simulink model "bla"  (R2023b)
settings: Solver=VariableStepAuto  StartTime=0.0  StopTime=10.0  RelTol=1e-3
undefined symbols (not defined in the file or in its folder): Bat, boost, ccm_mpp_reg_param, ccm_reg_param, Ci, dcm_mpp_reg_param, dcm_reg_param, m0_ccm, mppt_my3, pv_data, pv_eq, Ramp, sim_op, Tmfc, Ubat_CV_limit, Upv_ref
libraries: spsSeriesRLCBranchLib x5, spsCurrentMeasurementLib x2, spsVoltageMeasurementLib x2, spsControlledVoltageSourceLib x1, spsDiodeLib x1, spsControlledCurrentSourceLib x1, spsBistableLib x1, slpidlib x1, spsIdealSwitchLib x1
settings Model: Creator=teo  LastModifiedBy=teo

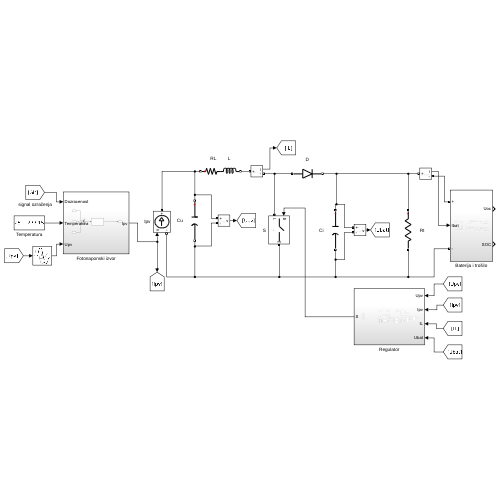
[thumbnail: Simulink's stored preview of the top-level diagram]
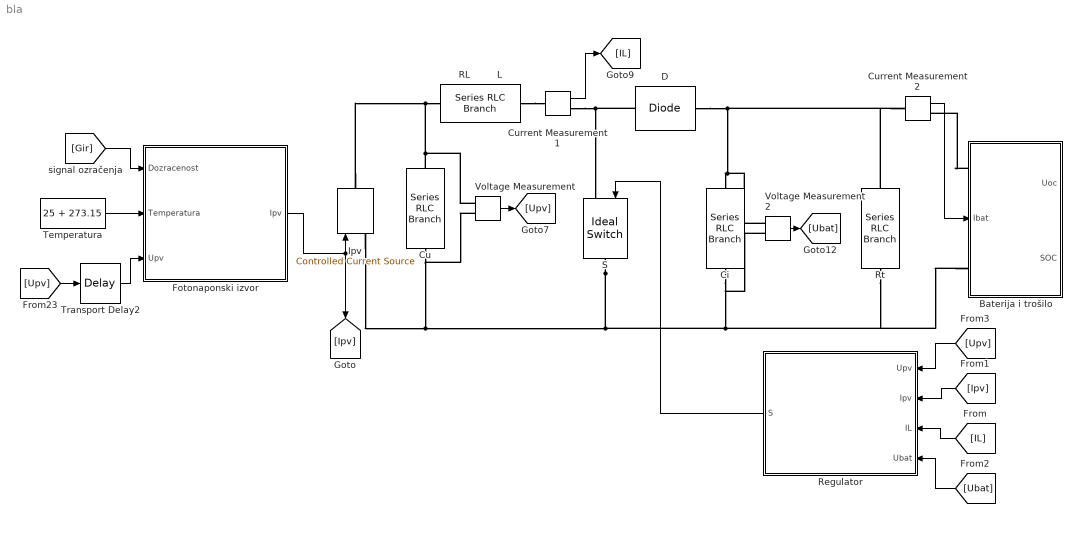
== system bla ==
  Baterija i trošilo : Subsystem
      settings: PortSchema="{\"entries\":[{\"content\":{\"sides\":[{\"content\":{\"connectorIds\":[\"LConn1\",\"In1\",\"LConn2\"]},\"type\":\"ConnectorPlacement.EquallySpacedRectSide\",\"uuid\":\"36a151cb-ade8-4d77-9227-5d94720a867f\"},{\"content\":{\"connectorIds\":[\"Out1\",\"Out2\"],\"side\":\"RIGHT\"},\"type\":\"ConnectorPlacement.EquallySpacedRectSide\",\"uuid\":\"e273b59b-5ac5-431a-9422-aa1eb85d6b42\"},{\"content\":{\"side\":\"TOP\"},\"type\":\"ConnectorPlacement.EquallySpacedRectSide\",\"uuid\":\"963da400-5a20-4c48-ad4c-e087b1b0be12\"}]},\"type\":\"ConnectorPlacement.EquallySpacedConnector\",\"uuid\":\"3f6c7281-abab-4595-a869-b172f12b4791\"}],\"packageUris\":[\"http://schema.mathworks.com/mf0/Connector/R2020b\"],\"version\":\"1.0\"}"
  Ci : spsSeriesRLCBranchLib/Series RLC Branch  LConnTagsString=__new0  RConnTagsString=__new0  BranchType=C  Resistance=0.001  Inductance=1e-3  SetiL0=off  InitialCurrent=0  Capacitance=boost.Ci  Setx0=on  InitialVoltage=sim_op.Ubat0  Measurements=None
  Cu : spsSeriesRLCBranchLib/Series RLC Branch  LConnTagsString=__new0  RConnTagsString=__new0  BranchType=C  Resistance=0.001  Inductance=1e-3  SetiL0=off  InitialCurrent=0  Capacitance=boost.Cu  Setx0=on  InitialVoltage=sim_op.Upv0  Measurements=None
  Current Measurement1 : spsCurrentMeasurementLib/Current Measurement  PhasorSimulation=off  OutputType=Complex  PSBequivalent=0
  Current Measurement2 : spsCurrentMeasurementLib/Current Measurement  PhasorSimulation=off  OutputType=Complex  PSBequivalent=0
  D : spsDiodeLib/Diode  Ron=0  Lon=0  Vf=0  IC=0  UseSnubber=0  Rs=0  Cs=0  Measurements=off
  Fotonaponski izvor : Subsystem
  Ipv : spsControlledCurrentSourceLib/Controlled Current Source  Initialize=on  Source_Type=DC  Amplitude=0  Phase=0  Frequency=0  Measurements=None
  RL         L : spsSeriesRLCBranchLib/Series RLC Branch  LConnTagsString=__new0  RConnTagsString=__new0  BranchType=RL  Resistance=boost.RL  Inductance=boost.L  SetiL0=off  InitialCurrent=stepp.ir01  Capacitance=1e-6  Setx0=off  InitialVoltage=0  Measurements=None
  Regulator : Subsystem
  Rt : spsSeriesRLCBranchLib/Series RLC Branch  LConnTagsString=__new0  RConnTagsString=__new0  BranchType=R  Resistance=boost.Rt  Inductance=1e-3  SetiL0=off  InitialCurrent=0  Capacitance=Ci  Setx0=off  InitialVoltage=0  Measurements=None
  S : spsIdealSwitchLib/Ideal Switch  Ron=0  Lon=0  IC=0  Rs=0  Cs=0  Measurements=off
  Temperatura : Constant  Value=25 + 273.15
  Transport Delay2 : TransportDelay  DelayTime=0.0001  BufferSize=4024
  Voltage Measurement : spsVoltageMeasurementLib/Voltage Measurement  PhasorSimulation=off  OutputType=Complex  PSBequivalent=0
  Voltage Measurement2 : spsVoltageMeasurementLib/Voltage Measurement  PhasorSimulation=off  OutputType=Complex  PSBequivalent=0
  wires:
  Voltage Measurement2/1 -> [Ubat]
  Current Measurement1/1 -> [IL]
  [Gir] -> Fotonaponski izvor/1(Dozracenost)
  Temperatura/1 -> Fotonaponski izvor/2(Temperatura)
  Regulator/1(S) -> S/1
  Fotonaponski izvor/1(Ipv) -> Ipv/1, [Ipv]
  [Upv] -> Transport Delay2/1
  Transport Delay2/1 -> Fotonaponski izvor/3(Upv)
  Voltage Measurement/1 -> [Upv]
  Current Measurement2/1 -> Baterija i trošilo/1(Ibat)
  [IL] -> Regulator/3(IL)
  [Ipv] -> Regulator/2(Ipv)
  [Ubat] -> Regulator/4(Ubat)
  [Upv] -> Regulator/1(Upv)
  connections:
  S/RConn1 -- Baterija i trošilo/LConn2 -- Rt/RConn1 -- Ci/RConn1 -- Voltage Measurement2/LConn2 -- Ipv/LConn1 -- Voltage Measurement/LConn2 -- Cu/RConn1
  D/RConn1 -- Current Measurement2/LConn1 -- Rt/LConn1 -- Voltage Measurement2/LConn1 -- Ci/LConn1
  Cu/LConn1 -- Voltage Measurement/LConn1 -- Ipv/RConn1 -- RL         L/LConn1
  Current Measurement1/RConn1 -- D/LConn1 -- S/LConn1
  Baterija i trošilo/LConn1 -- Current Measurement2/RConn1
  RL         L/RConn1 -- Current Measurement1/LConn1

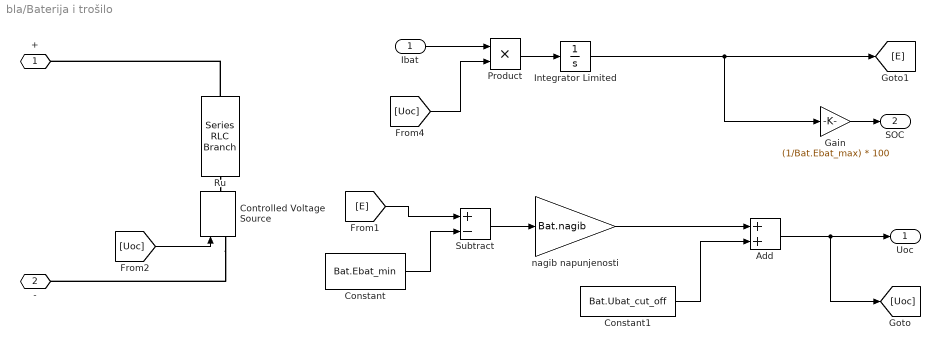
== system bla/Baterija i trošilo ==
  Ibat : Inport
  Add : Sum
  Constant : Constant  Value=Bat.Ebat_min
  Constant1 : Constant  Value=Bat.Ubat_cut_off
  Controlled Voltage Source : spsControlledVoltageSourceLib/Controlled Voltage Source  Initialize=on  Source_Type=DC  Amplitude=sim_op.Ubat0  Phase=0  Frequency=0  Measurements=None
  Gain : Gain  Gain=(1/Bat.Ebat_max) * 100
  Integrator Limited : Integrator  InitialCondition=sim_op.E0  LimitOutput=on  UpperSaturationLimit=Bat.Ebat_max  LowerSaturationLimit=Bat.Ebat_min
  Product : Product
  Ru : spsSeriesRLCBranchLib/Series RLC Branch  LConnTagsString=__new0  RConnTagsString=__new0  BranchType=R  Resistance=boost.Ru  Inductance=1e-3  SetiL0=off  InitialCurrent=0  Capacitance=Ci  Setx0=off  InitialVoltage=0  Measurements=None
  Subtract : Sum  Inputs=+-
  nagib napunjenosti : Gain  Gain=Bat.nagib
  + : PMIOPort  Side=Left
  - : PMIOPort  Port=2  Side=Left
  Uoc : Outport
  SOC : Outport  Port=2
  wires:
  Subtract/1 -> nagib napunjenosti/1
  Constant/1 -> Subtract/2
  nagib napunjenosti/1 -> Add/1
  Constant1/1 -> Add/2
  Integrator Limited/1 -> Gain/1, [E]
  [Uoc] -> Product/2
  Product/1 -> Integrator Limited/1
  Ibat/1 -> Product/1
  [E] -> Subtract/1
  [Uoc] -> Controlled Voltage Source/1
  Gain/1 -> SOC/1
  Add/1 -> Uoc/1, [Uoc]
  connections:
  Controlled Voltage Source/LConn1 -- -/RConn1
  Ru/RConn1 -- Controlled Voltage Source/RConn1
  Ru/LConn1 -- +/RConn1

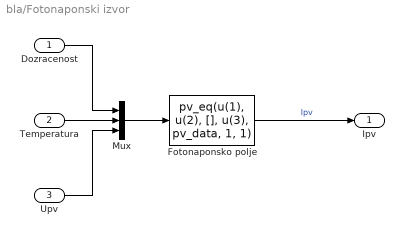
== system bla/Fotonaponski izvor ==
  Dozracenost : Inport
  Temperatura : Inport  Port=2
  Upv : Inport  Port=3
  Fotonaponsko polje : MATLABFcn  MATLABFcn=pv_eq(u(1), u(2), [], u(3), pv_data, 1, 1)  OutputDimensions=1
  Mux : Mux  Inputs=3
  Ipv : Outport
  wires:
  Fotonaponsko polje/1 -> Ipv/1  "Ipv"
  Mux/1 -> Fotonaponsko polje/1
  Dozracenost/1 -> Mux/1
  Temperatura/1 -> Mux/2
  Upv/1 -> Mux/3

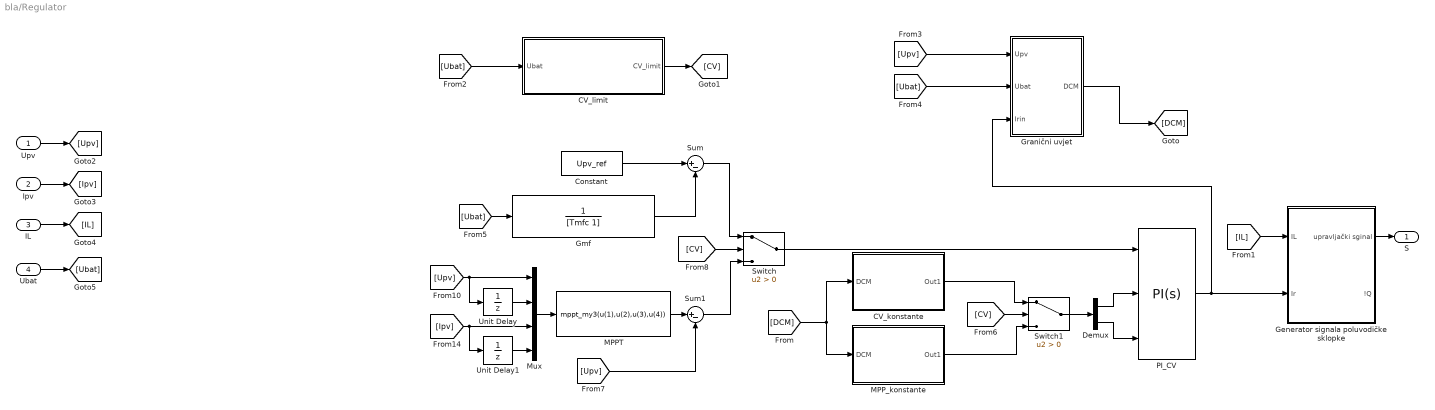
== system bla/Regulator ==
  Upv : Inport
  Ipv : Inport  Port=2
  IL : Inport  Port=3
  Ubat : Inport  Port=4
  CV_konstante : Subsystem
  CV_limit : Subsystem
  Constant : Constant  Value=Upv_ref
  Demux : Demux  Outputs=2
  Generator signala poluvodičke sklopke : Subsystem
  Gmf : TransferFcn  Numerator=1  Denominator=[Tmfc 1]
  Granični uvjet : Subsystem
  MPPT : MATLABFcn  MATLABFcn=mppt_my3(u(1),u(2),u(3),u(4))
  MPP_konstante : Subsystem
  Mux : Mux
  PI_CV : slpidlib/PID Controller  Controller=PI  Form=Parallel  TimeDomain=Continuous-time  UseExternalTs=off  SampleTime=-1  IntegratorMethod=Forward Euler  FilterMethod=Forward Euler  ControllerParametersSource=external  P=ccm_mpp_reg_param.KR  I=ccm_mpp_reg_param.KR/ccm_mpp_reg_param.Ti  UseKiTs=off  D=0  N=100  UseFilter=on  TunerSelectOption=Transfer Function Based (PID Tuner App)  InitialConditionSource=internal  InitialConditionForIntegrator=0  InitialConditionForFilter=0  DifferentiatorICPrevScaledInput=0  ExternalReset=none  TrackingMode=off  Kt=1  LimitOutput=on  SatLimitsSource=internal  UpperSaturationLimit=2  LowerSaturationLimit=-2  LinearizeAsGain=off  AntiWindupMode=clamping  Kb=1  LimitIntegrator=off  UpperIntegratorSaturationLimit=inf  LowerIntegratorSaturationLimit=-inf  POutMin=[]  POutMax=[]  IOutMin=[]  IOutMax=[]  DOutMin=[]  DOutMax=[]  NOutMin=[]  NOutMax=[]  SumOutMin=[]  SumOutMax=[]  SaturationOutMin=[]  SaturationOutMax=[]  PParamMin=[]  PParamMax=[]  IParamMin=[]  IParamMax=[]  DParamMin=[]  DParamMax=[]  NParamMin=[]  NParamMax=[]  KbParamMin=[]  KbParamMax=[]  KtParamMin=[]  KtParamMax=[]  KbOutMin=[]  KbOutMax=[]  KtOutMin=[]  KtOutMax=[]  IntegratorOutMin=[]  IntegratorOutMax=[]  FilterOutMin=[]  FilterOutMax=[]  SumI1OutMin=[]  SumI1OutMax=[]  SumI2OutMin=[]  SumI2OutMax=[]  SumI3OutMin=[]  SumI3OutMax=[]  SumI4OutMin=[]  SumI4OutMax=[]  SumDOutMin=[]  SumDOutMax=[]  DifferentiatorOutMin=[]  DifferentiatorOutMax=[]  FilterDiffOutCoefMin=[]  FilterDiffOutCoefMax=[]  ReciprocalOutMin=[]  ReciprocalOutMax=[]  SumDenOutMin=[]  SumDenOutMax=[]  SumNumOutMin=[]  SumNumOutMax=[]  DivideOutMin=[]  DivideOutMax=[]  UdiffTsProdOutMin=[]  UdiffTsProdOutMax=[]  NTsProdOutMin=[]  NTsProdOutMax=[]  UintegralTsProdOutMin=[]  UintegralTsProdOutMax=[]  UngainTsProdOutMin=[]  UngainTsProdOutMax=[]  ClampingZeroOutDataTypeStr=Inherit: Inherit via back propagation  ClampingZeroOutMin=[]  ClampingZeroOutMax=[]  FilterDenConstantOutDataTypeStr=Inherit: Inherit via back propagation  FilterDenConstantOutMin=[]  FilterDenConstantOutMax=[]  PCopyOutDataTypeStr=Inherit: Inherit via back propagation  PCopyOutMin=[]  PCopyOutMax=[]  NCopyOutDataTypeStr=Inherit: Inherit via back propagation  NCopyOutMin=[]  NCopyOutMax=[]  IntegratorContinuousStateAttributes=''  IntegratorStateMustResolveToSignalObject=off  IntegratorRTWStateStorageClass=Auto  FilterContinuousStateAttributes=''  FilterStateMustResolveToSignalObject=off  FilterRTWStateStorageClass=Auto  ParallelPVariant=ExternalParameters  IdealPVariant=Disabled  IVariant=ExternalParameters  DVariant=Disabled  IntegratorVariant=Continuous  SatVariant=Enabled  AWVariant=ContClampingParallel  PCopyVariant=Disabled  TRVariant=Disabled  FdbkBlocksVariant=Forward  IdealPFdbkVariant=Disabled  SatFdbkVariant=Disabled  DerivativeFilterVariant=Disabled  NVariant=Disabled  NCopyVariant=Disabled_SignalSpec  FilterICVariant=Disabled  IntegratorICVariant=InternalICs  ExternalResetVariant=Disabled  TRSumVariant=Passthrough  SumFdbkVariant=Disabled  SumVariant=Sum_PI  TsampFilterVariant=InternalTs  TsampNgainVariant=Passthrough  TsampIntegralVariant=Disabled_SignalSpec  ExternalSaturationOutDataTypeStr=Inherit: Same as second input
  Sum : Sum  Inputs=|+-
  Sum1 : Sum  Inputs=|+-
  Switch : Switch  Criteria=u2 > Threshold  SaturateOnIntegerOverflow=off  InputSameDT=off
  Switch1 : Switch  Criteria=u2 > Threshold  SaturateOnIntegerOverflow=off  InputSameDT=off
  Unit Delay : UnitDelay  SampleTime=-1  HasFrameUpgradeWarning=on
  Unit Delay1 : UnitDelay  SampleTime=-1  HasFrameUpgradeWarning=on
  S : Outport
  wires:
  Switch1/1 -> Demux/1
  Demux/1 -> PI_CV/2
  Demux/2 -> PI_CV/3
  Generator signala poluvodičke sklopke/1(upravljački sginal) -> S/1
  Upv/1 -> [Upv]
  Ipv/1 -> [Ipv]
  Ubat/1 -> [Ubat]
  IL/1 -> [IL]
  Granični uvjet/1(DCM) -> [DCM]
  [Ubat] -> Granični uvjet/2(Ubat)
  PI_CV/1 -> Generator signala poluvodičke sklopke/2(Ir), Granični uvjet/3(Irin)
  [IL] -> Generator signala poluvodičke sklopke/1(IL)
  [Ubat] -> Gmf/1
  Constant/1 -> Sum/1
  Gmf/1 -> Sum/2
  Unit Delay1/1 -> Mux/4
  Unit Delay/1 -> Mux/2
  MPPT/1 -> Sum1/1
  [Upv] -> Sum1/2
  Mux/1 -> MPPT/1
  [Upv] -> Unit Delay/1, Mux/1
  [Ipv] -> Unit Delay1/1, Mux/3
  CV_konstante/1(Out1) -> Switch1/1
  MPP_konstante/1(Out1) -> Switch1/3
  [DCM] -> MPP_konstante/1(DCM), CV_konstante/1(DCM)
  [Ubat] -> CV_limit/1(Ubat)
  [Upv] -> Granični uvjet/1(Upv)
  CV_limit/1(CV_limit) -> [CV]
  [CV] -> Switch1/2
  [CV] -> Switch/2
  Switch/1 -> PI_CV/1
  Sum/1 -> Switch/1
  Sum1/1 -> Switch/3

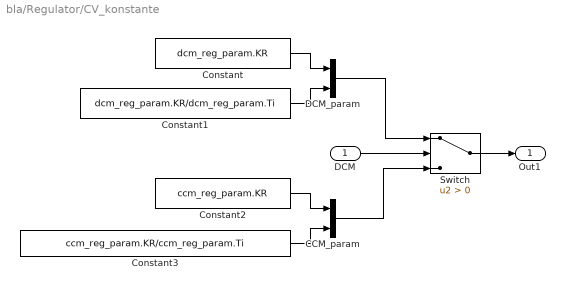
== system bla/Regulator/CV_konstante ==
  DCM : Inport
  CCM_param : Mux  Inputs=2
  Constant : Constant  Value=dcm_reg_param.KR
  Constant1 : Constant  Value=dcm_reg_param.KR/dcm_reg_param.Ti
  Constant2 : Constant  Value=ccm_reg_param.KR
  Constant3 : Constant  Value=ccm_reg_param.KR/ccm_reg_param.Ti
  DCM_param : Mux  Inputs=2
  Switch : Switch  Criteria=u2 > Threshold  SaturateOnIntegerOverflow=off  InputSameDT=off
  Out1 : Outport
  wires:
  Constant/1 -> DCM_param/1
  Constant1/1 -> DCM_param/2
  DCM_param/1 -> Switch/1
  Constant2/1 -> CCM_param/1
  Constant3/1 -> CCM_param/2
  CCM_param/1 -> Switch/3
  Switch/1 -> Out1/1
  DCM/1 -> Switch/2

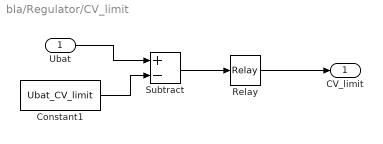
== system bla/Regulator/CV_limit ==
  Ubat : Inport
  Constant1 : Constant  Value=Ubat_CV_limit
  Relay : Relay  OnSwitchValue=0  OffSwitchValue=-0.5
  Subtract : Sum  Inputs=+-
  CV_limit : Outport
  wires:
  Constant1/1 -> Subtract/2
  Subtract/1 -> Relay/1
  Relay/1 -> CV_limit/1
  Ubat/1 -> Subtract/1

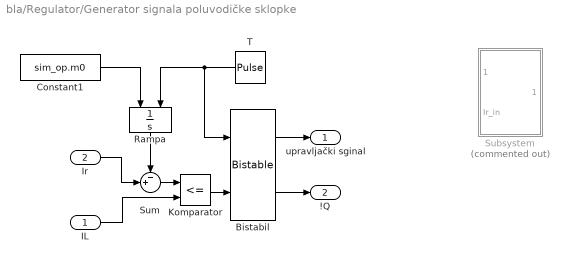
== system bla/Regulator/Generator signala poluvodičke sklopke ==
  IL : Inport
  Ir : Inport  Port=2
  Bistabil : spsBistableLib/Bistable  Qpriority=Set  ic=0  Ts=0
      settings: LibrarySourceBlock=sps_lib/Control/Bistable
  Constant1 : Constant  Value=sim_op.m0
  Komparator : RelationalOperator  Operator=<=  OutDataTypeStr=boolean  RndMeth=Simplest  InputSameDT=off
  Rampa : Integrator  ExternalReset=rising
  Subsystem : Subsystem  Commented=on
  Sum : Sum  Inputs=-+|
  T : DiscretePulseGenerator  PulseType=Time based  Period=boost.T
  upravljački sginal : Outport
  !Q : Outport  Port=2
  wires:
  Komparator/1 -> Bistabil/2
  Bistabil/2 -> !Q/1
  Bistabil/1 -> upravljački sginal/1
  IL/1 -> Komparator/2
  Sum/1 -> Komparator/1
  Ir/1 -> Sum/2
  Rampa/1 -> Sum/1
  T/1 -> Bistabil/1, Rampa/2
  Constant1/1 -> Rampa/1

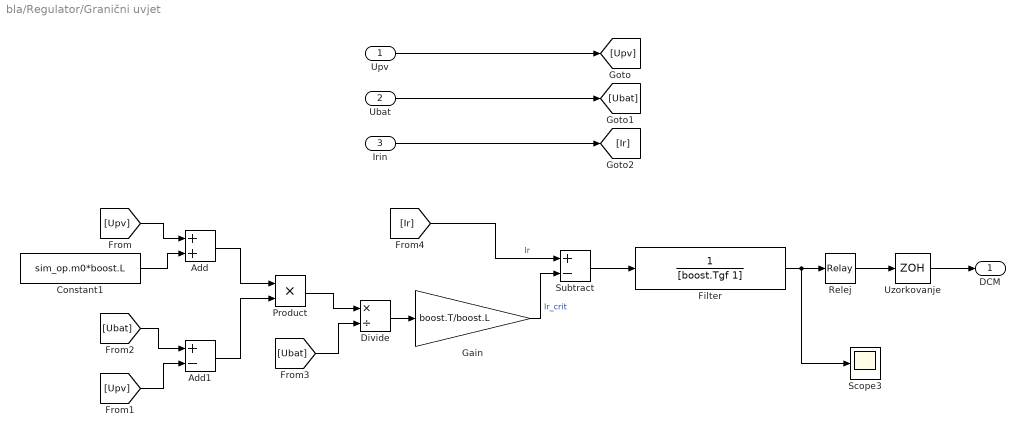
== system bla/Regulator/Granični uvjet ==
  Upv : Inport
  Ubat : Inport  Port=2
  Irin : Inport  Port=3
  Add : Sum
  Add1 : Sum  Inputs=+-
  Constant1 : Constant  Value=sim_op.m0*boost.L
  Divide : Product  Inputs=*/
  Filter : TransferFcn  Numerator=1  Denominator=[boost.Tgf 1]
  Gain : Gain  Gain=boost.T/boost.L
  Product : Product
  Relej : Relay  OnSwitchValue=0.01  OffSwitchValue=-0.01  OnOutputValue=0  OffOutputValue=1
  Scope3 : Scope
  Subtract : Sum  Inputs=+-
  Uzorkovanje : ZeroOrderHold  SampleTime=0.001
  DCM : Outport
  wires:
  Product/1 -> Divide/1
  Constant1/1 -> Add/2
  Add/1 -> Product/1
  Add1/1 -> Product/2
  Divide/1 -> Gain/1
  [Upv] -> Add/1
  [Upv] -> Add1/2
  [Ubat] -> Add1/1
  [Ubat] -> Divide/2
  Gain/1 -> Subtract/2  "Ir_crit"
  [Ir] -> Subtract/1  "Ir"
  Relej/1 -> Uzorkovanje/1
  Upv/1 -> [Upv]
  Ubat/1 -> [Ubat]
  Irin/1 -> [Ir]
  Subtract/1 -> Filter/1
  Filter/1 -> Scope3/1, Relej/1
  Uzorkovanje/1 -> DCM/1

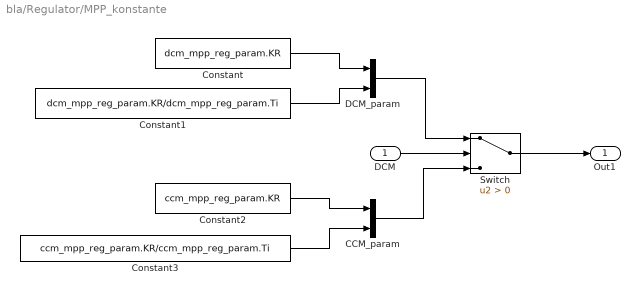
== system bla/Regulator/MPP_konstante ==
  DCM : Inport
  CCM_param : Mux  Inputs=2
  Constant : Constant  Value=dcm_mpp_reg_param.KR
  Constant1 : Constant  Value=dcm_mpp_reg_param.KR/dcm_mpp_reg_param.Ti
  Constant2 : Constant  Value=ccm_mpp_reg_param.KR
  Constant3 : Constant  Value=ccm_mpp_reg_param.KR/ccm_mpp_reg_param.Ti
  DCM_param : Mux  Inputs=2
  Switch : Switch  Criteria=u2 > Threshold  SaturateOnIntegerOverflow=off  InputSameDT=off
  Out1 : Outport
  wires:
  DCM_param/1 -> Switch/1
  CCM_param/1 -> Switch/3
  Switch/1 -> Out1/1
  DCM/1 -> Switch/2
  Constant/1 -> DCM_param/1
  Constant1/1 -> DCM_param/2
  Constant2/1 -> CCM_param/1
  Constant3/1 -> CCM_param/2

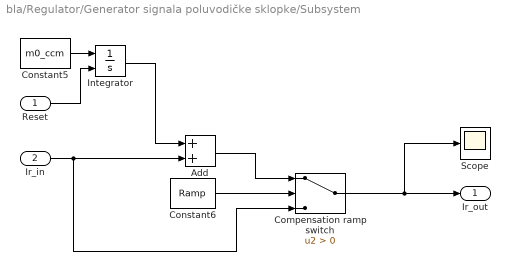
== system bla/Regulator/Generator signala poluvodičke sklopke/Subsystem ==
  Reset : Inport
  Ir_in : Inport  Port=2
  Add : Sum
  Compensation ramp switch : Switch  Criteria=u2 > Threshold  SaturateOnIntegerOverflow=off  InputSameDT=off
  Constant5 : Constant  Value=m0_ccm
  Constant6 : Constant  Value=Ramp
  Integrator : Integrator  ExternalReset=rising
  Scope : Scope
  Ir_out : Outport
  wires:
  Constant5/1 -> Integrator/1
  Integrator/1 -> Add/1
  Add/1 -> Compensation ramp switch/1
  Reset/1 -> Integrator/2
  Compensation ramp switch/1 -> Scope/1, Ir_out/1
  Constant6/1 -> Compensation ramp switch/2
  Ir_in/1 -> Compensation ramp switch/3, Add/2
